simulink model "MC_R2_SFC_RELOJ_sin_antisway"  (R2025b)
settings: Solver=ode23t  StartTime=0.0  StopTime=600  MaxStep=T_s  RelTol=1e-4
InitFcn:
  | addpath(fileparts(get_param(bdroot,'FileName')),'-begin');
  | run(fullfile(fileparts(get_param(bdroot,'FileName')),'definir_buses_variadores.m'));
  | run(fullfile(fileparts(get_param(bdroot,'FileName')),'parametros_ganancias_cascada_29072026.m'));
  | run(fullfile(fileparts(get_param(bdroot,'FileName')),'configurar_modelo_final_hmi.m'));
  | run(fullfile(fileparts(get_param(bdroot,'FileName')),'configurar_parametros_variadores.m'));
  | Pvis.Ts_viz=0.04;Pvis.hmi.testDriver=@operador_medio_ciclo;
StopFcn:
  | cerrar_video_ensayo;
values from neighbouring files (symbols this model uses):
  MC_FF = struct('Ts',T_s,'gravity',g,'r_td',r_td,'i_t',i_t,'M_EQt',M_EQt,   'b_EQt',b_EQt,'Kx',K_x_cas,'Kp',K_pv_cas,'Ki',K_iv_cas,   'vmax',v_tmax,'amax',dv_tmax,'Imax',dv_tmax/K_iv_cas,   'r_hd',r_hd,'i_h',i_h,'M_EQh',M_EQh,'b_EQh',b_EQh,   'Khp',K_hp,'Khi',K_hi,'Khd',K_hd,'length0',l_hi,'swayOnTime',T_SW_on,   'swayFFRate',0.25,'observerWn',40.0,'observerZeta',1.0)    [configurar_parametros_variadores.m]
undefined symbols (not defined in the file or in its folder): b_cx, b_cy, b_hb, b_hEb, b_heq, b_t, b_tb, b_teq, b_tw, b_wu, g, H_c, HMI, i_h, i_t, J_heq, J_teq, K_cy, K_tw, k_wu, L_h0, l_hi, M_c_profile, M_s, M_t, nLevels0, omega_hmRATED, r_hd, r_td, slotBlock, T_hbMax, T_hEbMax, T_hmMax, T_s, T_s1, T_tbMax, T_tmMax, tau_hm, tau_tm, traj_duration, traj_x_start, traj_x_target, v_hmaxLoaded, v_hmaxUnloaded, x_tmax, x_tmin, Y_c0, Y_t0, Zbase
libraries: simulink x1, aerolibanimutils x1
(part 3 of 3)

== system MC_R2_SFC_RELOJ_sin_antisway/Planta/Subsistema carro/Modelo Freno Operacion Carro ==
  BRK_t : Inport
  omega_tm : Inport  Port=2
  Constant : Constant  Value=0
  Gain : Gain  Gain=-b_tb
  Saturation : Saturate  UpperLimit=T_tbMax  LowerLimit=-T_tbMax
  Switch : Switch  Criteria=u2 > Threshold  SaturateOnIntegerOverflow=off  InputSameDT=off
  T_tb : Outport
  wires:
  Saturation/1 -> Switch/3
  omega_tm/1 -> Gain/1
  Switch/1 -> T_tb/1
  Gain/1 -> Saturation/1
  Constant/1 -> Switch/1
  BRK_t/1 -> Switch/2

== system MC_R2_SFC_RELOJ_sin_antisway/Planta/Subsistema carro/Modulador de Torque Motor Drive Carro ==
  T_tm* : Inport
  Diferencia torque saturacion : Sum  Inputs=+-
  Gain : Gain  Gain=1/tau_tm
  Integrator : Integrator
  Saturation : Saturate  UpperLimit=T_tmMax  LowerLimit=-T_tmMax
  Sum : Sum  Inputs=|+-
  T_tm : Outport
  Delta torque limite : Outport  Port=2
  wires:
  Integrator/1 -> Sum/2, T_tm/1
  Gain/1 -> Integrator/1
  Sum/1 -> Gain/1
  Saturation/1 -> Sum/1, Diferencia torque saturacion/1  "T_tmlim*"
  T_tm*/1 -> Saturation/1, Diferencia torque saturacion/2
  Diferencia torque saturacion/1 -> Delta torque limite/1

== system MC_R2_SFC_RELOJ_sin_antisway/Planta/Subsistema izaje/Calculo longitud l_h ==
  note: $\dot{l}_h(t)=-\frac{r_{hd}}{2}\omega_{hd}(t)$
  omega_hd : Inport
  Gain : Gain  Gain=-r_hd/2
  Integrator : Integrator  InitialCondition=l_hi
  l_h : Outport
  dl_h : Outport  Port=2
  wires:
  Integrator/1 -> l_h/1  "l_h"
  omega_hd/1 -> Gain/1
  Gain/1 -> dl_h/1, Integrator/1  "dl_h"

== system MC_R2_SFC_RELOJ_sin_antisway/Planta/Subsistema izaje/Dinamica Tambor Izaje ==
  T_hEb : Inport
  T_hm : Inport  Port=2
  F_hw : Inport  Port=3
  T_hb : Inport  Port=4
  Gain1 : Gain  Gain=r_hd
  Gain2 : Gain  Gain=1/i_h
  Gain3 : Gain  Gain=1/J_heq
  Gain4 : Gain  Gain=b_heq
  Gain5 : Gain  Gain=1/i_h
  Integrator2 : Integrator
  Integrator3 : Integrator
  Sum1 : Sum  Inputs=+++--
  theta_hd : Outport
  omega_hd : Outport  Port=2
  wires:
  Gain3/1 -> Integrator2/1  "ddtheta_hd"
  Integrator2/1 -> omega_hd/1, Gain4/1, Integrator3/1  "omega_hd"
  Sum1/1 -> Gain3/1
  T_hb/1 -> Sum1/2
  T_hEb/1 -> Gain5/1  "T_hEb"
  Gain4/1 -> Sum1/5
  Gain5/1 -> Sum1/3
  T_hm/1 -> Sum1/1
  F_hw/1 -> Gain1/1
  Gain1/1 -> Gain2/1  "T_hdl"
  Gain2/1 -> Sum1/4
  Integrator3/1 -> theta_hd/1  "theta_hd"

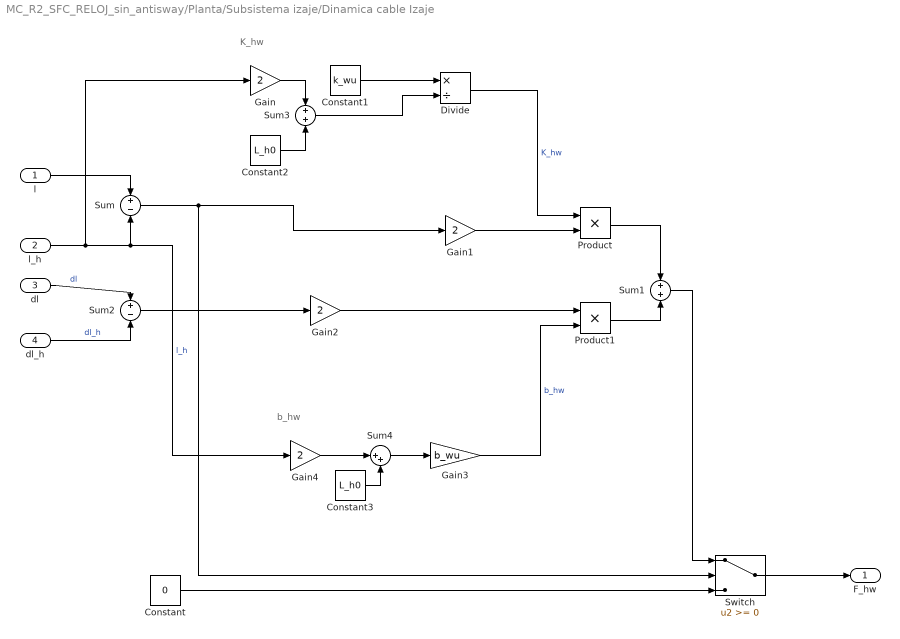
== system MC_R2_SFC_RELOJ_sin_antisway/Planta/Subsistema izaje/Dinamica cable Izaje ==
  note: b_hw
  note: K_hw
  l : Inport
  l_h : Inport  Port=2
  dl : Inport  Port=3
  dl_h : Inport  Port=4
  Constant : Constant  Value=0
  Constant1 : Constant  Value=k_wu
  Constant2 : Constant  Value=L_h0
  Constant3 : Constant  Value=L_h0
  Divide : Product  Inputs=*/
  Gain{,1..2,4} (4 alike) : Gain  Gain=2
  Gain3 : Gain  Gain=b_wu
  Product : Product
  Product1 : Product
  Sum : Sum  Inputs=+-
  Sum1 : Sum
  Sum2 : Sum  Inputs=+-
  Sum3 : Sum
  Sum4 : Sum  Inputs=|++
  Switch : Switch  SaturateOnIntegerOverflow=off  InputSameDT=off
  F_hw : Outport
  wires:
  Constant/1 -> Switch/3
  l/1 -> Sum/1
  l_h/1 -> Gain4/1, Sum/2, Gain/1  "l_h"
  Sum/1 -> Switch/2, Gain1/1
  Switch/1 -> F_hw/1
  Sum1/1 -> Switch/1
  Gain1/1 -> Product/2
  Product/1 -> Sum1/1
  Divide/1 -> Product/1  "K_hw"
  Gain3/1 -> Product1/2  "b_hw"
  dl/1 -> Sum2/1  "dl"
  dl_h/1 -> Sum2/2  "dl_h"
  Sum2/1 -> Gain2/1
  Gain2/1 -> Product1/1
  Product1/1 -> Sum1/2
  Sum3/1 -> Divide/2
  Constant1/1 -> Divide/1
  Constant2/1 -> Sum3/2
  Gain/1 -> Sum3/1
  Gain4/1 -> Sum4/1
  Sum4/1 -> Gain3/1
  Constant3/1 -> Sum4/2

== system MC_R2_SFC_RELOJ_sin_antisway/Planta/Subsistema izaje/Modelo Freno Emergencia de Izaje(Eje lento) ==
  omega_hd : Inport
  BRK_hE : Inport  Port=2
  Constant : Constant  Value=0
  Gain : Gain  Gain=-b_hEb
  Saturation : Saturate  UpperLimit=T_hEbMax  LowerLimit=-T_hEbMax
  Switch : Switch  Criteria=u2 > Threshold  SaturateOnIntegerOverflow=off  InputSameDT=off
  T_hEb : Outport
  wires:
  Saturation/1 -> Switch/3
  omega_hd/1 -> Gain/1
  Switch/1 -> T_hEb/1
  Gain/1 -> Saturation/1
  Constant/1 -> Switch/1
  BRK_hE/1 -> Switch/2

== system MC_R2_SFC_RELOJ_sin_antisway/Planta/Subsistema izaje/Modelo Freno Operacion de Izaje(Eje Rapido) ==
  BRK_h : Inport
  omega_hm : Inport  Port=2
  Constant : Constant  Value=0
  Gain : Gain  Gain=-b_hb
  Saturation : Saturate  UpperLimit=T_hbMax  LowerLimit=-T_hbMax
  Switch : Switch  Criteria=u2 > Threshold  SaturateOnIntegerOverflow=off  InputSameDT=off
  T_hb : Outport
  wires:
  Saturation/1 -> Switch/3
  omega_hm/1 -> Gain/1
  Switch/1 -> T_hb/1
  Gain/1 -> Saturation/1
  Constant/1 -> Switch/1
  BRK_h/1 -> Switch/2

== system MC_R2_SFC_RELOJ_sin_antisway/Planta/Subsistema izaje/Modulador de Torque Motor Drive Izaje ==
  T_hm* : Inport
  omega_hm : Inport  Port=2
  Calculo Torque Limite : Subsystem
  Gain : Gain  Gain=1/tau_hm
  Gain1 : Gain  Gain=-1
  Integrator : Integrator
  Saturation Dynamic : simulink/Discontinuities/Saturation Dynamic  OutMin=[]  OutMax=[]  OutDataTypeStr=Inherit: Same as second input  OutDataType=fixdt(1, 16)  OutScaling=2^-10  DoSatur=off
  Sum : Sum  Inputs=|+-
  T_hm : Outport
  wires:
  Gain/1 -> Integrator/1
  Sum/1 -> Gain/1
  Integrator/1 -> T_hm/1, Sum/2
  Saturation Dynamic/1 -> Sum/1  "Thm_sat"
  T_hm*/1 -> Saturation Dynamic/2
  omega_hm/1 -> Calculo Torque Limite/1(omega_hm)
  Calculo Torque Limite/1(T_hmMax) -> Gain1/1, Saturation Dynamic/1
  Gain1/1 -> Saturation Dynamic/3

== system MC_R2_SFC_RELOJ_sin_antisway/Planta/Subsistema izaje/Modulador de Torque Motor Drive Izaje/Calculo Torque Limite ==
  omega_hm : Inport
  Abs omega : Abs  SaturateOnIntegerOverflow=off
  Constant2 : Constant
  Divide : Product  Inputs=*/
  Gain1 : Gain  Gain=T_hmMax
  Min : MinMax  Inputs=2
  Proteccion omega cero : Saturate  UpperLimit=inf  LowerLimit=1e-6
  Square : Math  Operator=square
  omega_hmRATED : Constant  Value=omega_hmRATED
  T_hmMax : Outport
  wires:
  omega_hmRATED/1 -> Divide/1
  Gain1/1 -> T_hmMax/1  "T_hmMax"
  Min/1 -> Gain1/1
  Constant2/1 -> Min/2
  Square/1 -> Min/1
  Divide/1 -> Square/1
  omega_hm/1 -> Abs omega/1
  Abs omega/1 -> Proteccion omega cero/1
  Proteccion omega cero/1 -> Divide/2

== stateflow chart MC_R2_SFC_RELOJ_sin_antisway/PICK // PLACE ==
  state INICIO
    entry:
    evento_cambio = false;
    tipo_evento = 0;
    slot_evento = -1;
    slot_mem = -1;
    carga_tomada = TLK;
  state VACIO1
    during:
    evento_cambio = false;
    tipo_evento = 0;
    slot_evento = -1;
    carga_tomada = 0;
  state PRE_PLACE
    during:
    evento_cambio = false;
    tipo_evento = 0;
    slot_evento = -1;
    carga_tomada = 1;
  state CARGADO1
    during:
    evento_cambio = false;
    tipo_evento = 0;
    slot_evento = -1;
    carga_tomada = 1;
  state PRE_PICK
    during:
    evento_cambio = false;
    tipo_evento = 0;
    slot_evento = -1;
    carga_tomada = 0;
  (default) -> ? [commented out]
  (default) -> ? [commented out] : [slot_ok && TLK == 1 && tension && ~contacto && v_yl > -0.05]{slot_evento = k_slot;}
  (default) -> ? [commented out] : [slot_ok && TLK == 0 && ~tension && contacto && abs(v_yl) < 0.05]{slot_evento = k_slot;}
  (default) -> ? [commented out] : [true]
  (default) -> INICIO
  INICIO -> VACIO1 [order 1] : [TLK==0]
  INICIO -> CARGADO1 [order 2] : [TLK ==1]
  PRE_PLACE -> VACIO1 [order 2] : [slot_ok && TLK == 0 && contacto]{evento_cambio = true; tipo_evento = 2; slot_evento = slot_mem;}
  CARGADO1 -> PRE_PLACE : [slot_ok && TLK == 1 && contacto && abs(v_yl) < 0.05]{slot_mem = k_slot;}
  PRE_PICK -> VACIO1 [order 1] : [~slot_ok || (~contacto && TLK == 0)]{slot_mem = -1;}
  PRE_PLACE -> CARGADO1 [order 1] : [TLK == 1 && tension && ~contacto && v_yl > 0.05]{slot_mem = -1;}
  VACIO1 -> PRE_PICK : [slot_ok && contacto && TLK == 0]{slot_mem = k_slot;}
  PRE_PICK -> CARGADO1 [order 2] : [slot_ok && TLK == 1 && tension && ~contacto && v_yl > 0.05]{evento_cambio = true; tipo_evento = 1; slot_evento = slot_mem;}
  data: TLK input; k_slot input; slot_ok input; v_yl input; evento_cambio output; tipo_evento output; slot_evento output int32; contacto input; tension input; slot_mem local int32; carga_tomada output

== matlab function MC_R2_SFC_RELOJ_sin_antisway/Histeresis_F_hw ==
  data: F_hw input; tension output
function tension = tension_hist_Fhw(F_hw)
% Histeresis física para detectar "cable cargado" a partir de F_hw [N].
% Basada en fracciones del peso mínimo (spreader + contenedor vacío).

% --- Parámetros físicos ---
g = 9.81;
M_s    = 15000;   % kg
M_cmin = 2000;    % kg

Wmin = (M_s + M_cmin) * g;     % N  ~ 167 kN

% --- Umbrales con histéresis ---
Fhw_on  = 0.21 * Wmin;         % ~ 35 kN (cable claramente cargado)
Fhw_off = 0.09 * Wmin;         % ~ 15 kN (cable claramente descargado)

% --- Estado persistente ---
persistent t
if isempty(t)
    t = false;
end

% --- Lógica de histéresis ---
if ~t
    if F_hw > Fhw_on
        t = true;
    end
else
    if F_hw < Fhw_off
        t = false;
    end
end

tension = t;
end

== matlab function MC_R2_SFC_RELOJ_sin_antisway/Histeresis_contacto ==
  data: F_cy input; contacto output
function contacto = contacto_hist_Fcy(F_cy)
% Histeresis física para detectar contacto a partir de F_cy [N].
% Basada en fracciones del peso mínimo (spreader + contenedor vacío).

% --- Parámetros físicos ---
g = 9.81;
M_s    = 15000;   % kg
M_cmin = 2000;    % kg

Wmin = (M_s + M_cmin) * g;     % N  ~ 167 kN

% --- Umbrales con histéresis ---
Fcy_on  = 0.03  * Wmin;        % ~ 5 kN (entra a contacto)
Fcy_off = 0.012 * Wmin;        % ~ 2 kN (sale de contacto)

% --- Estado persistente ---
persistent c
if isempty(c)
    c = false;
end

% --- Lógica de histéresis ---
if ~c
    if F_cy > Fcy_on
        c = true;
    end
else
    if F_cy < Fcy_off
        c = false;
    end
end

contacto = c;
end

== matlab function MC_R2_SFC_RELOJ_sin_antisway/slot_x_l ==
  data: x_l input; k_slot output; slot_ok output; slotBlock input
function [k_slot, slot_ok] = xl_a_slot(x_l, slotBlock)
%#codegen

x0 = -30.0;
slotWidth = 2.44;
Nslots = int32(length(slotBlock));

k = int32(1) + int32(floor((x_l - x0) / slotWidth));

if (k < 1) || (k > Nslots)
    k_slot = int32(-1);
    slot_ok = false;
else
    k_slot = k;
    slot_ok = ~slotBlock(k_slot);
end

end

== matlab function MC_R2_SFC_RELOJ_sin_antisway/Actualizar_Yc/update_perfil_std ==
  data: nLevels input; nLevels_new output; tipo_evento input; slot_evento input; Y_c output; Zbase input; slotBlock input; h_std input
function [nLevels_new, Y_c] = update_profile_std(nLevels, tipo_evento, slot_evento, Zbase, slotBlock, h_std)
% UPDATE_PROFILE_STD
% Actualiza el perfil discreto de obstáculos.
% Convención:
%   Y_c(k)       = altura absoluta física del tope del obstáculo.
%   nLevels(k)  = cantidad de containers en el slot k.
%   Zbase(k)    = base física absoluta del slot k.
%   slotBlock(k)= true si el slot no es operable.
%
% tipo_evento:
%   0 = NONE
%   1 = PICK
%   2 = PLACE

Nslots = int32(length(nLevels));

nLevels_new = nLevels;

slot = int32(slot_evento);

slot_ok = (slot >= 1) && (slot <= Nslots) && (~slotBlock(slot));

if slot_ok
    if tipo_evento == 1
        nLevels_new(slot) = max(nLevels_new(slot) - 1, 0);

    elseif tipo_evento == 2
        nLevels_new(slot) = nLevels_new(slot) + 1;
    end

end

Y_c = Zbase + double(nLevels_new) * h_std;

% En slots bloqueados no se codifica bloqueo dentro de Y_c.
% Se deja una altura neutral coherente con Zbase.
Y_c(slotBlock) = Zbase(slotBlock);

end

== stateflow chart MC_R2_SFC_RELOJ_sin_antisway/Trayectoria ==
  settings: updateMethod=DISCRETE  sampleTime=T_s  description=Generador parametrico de septimo orden. Mantiene continuas x, v, a y jerk y conserva la interfaz original.
  state Perfil_suave
    during:
    tau = elapsed/traj_duration;
    if tau > 1
    tau = 1;
    end
    delta_x = traj_x_target-traj_x_start;
    sigma = 35*tau^4-84*tau^5+70*tau^6-20*tau^7;
    dsigma = 140*tau^3-420*tau^4+420*tau^5-140*tau^6;
    d2sigma = 420*tau^2-1680*tau^3+2100*tau^4-840*tau^5;
    d3sigma = 840*tau-5040*tau^2+8400*tau^3-4200*tau^4;
    x_act = traj_x_start+delta_x*sigma;
    v_act = delta_x*dsigma/traj_duration;
    a_act = delta_x*d2sigma/(traj_duration^2);
    j_act = delta_x*d3sigma/(traj_duration^3);
    elapsed = elapsed+T_s;
  state Objetivo
    entry:
    x_act = traj_x_target;
    v_act = 0;
    a_act = 0;
    j_act = 0;
  state Esperando
    entry:
    elapsed = 0;
    x_act = traj_x_start;
    v_act = 0;
    a_act = 0;
    j_act = 0;
  (default) -> Esperando
  Perfil_suave -> Objetivo : [elapsed >= traj_duration]
  Esperando -> Perfil_suave : [iniciar == 1]
  data: j_k function_output; v_max function_input; a_max function_input; j_max function_input; j_min function_input; v_k function_input; a_k function_input; d_k function_output; fa_min function_input; a_min function_input; j_max function_input; j_min function_input; a_k function_input; a_1 function_input; v_k function_input; v_1 function_input; T_j2a function_output; T_j2b function_output; T_d function_output; j_k function_output; j_min function_input; j_max function_input; k function_input; k_d function_input; T_s function_input; T_d function_input; T_j2a function_input; T_j2b function_input; iniciar input double =0; v_act output double =0; x_act output double =0; a_act output double =0; j_act output double =0; traj_x_start parameter double; traj_x_target parameter double; traj_duration parameter double; T_s parameter double; elapsed local double =0; tau local double =0; delta_x local double =0; sigma local double =0; dsigma local double =0; d2sigma local double =0; d3sigma local double =0
  function j_k=calculo_jerk(v_max, a_max, j_max, j_min, v_k, a_k):
    | function j_k=calculo_jerk(v_max, a_max, j_max, j_min, v_k, a_k)
    | 
    | if ((v_k-(a_k^2)/(2*j_min))<v_max)&&(a_k<a_max)
    |     j_k = j_max;
    | elseif ((v_k-(a_k^2)/(2*j_min))<v_max)&&(a_k>=a_max)
    |     j_k = 0;
    | elseif ((v_k-(a_k^2)/(2*j_min))>=v_max)&&(a_k>0)
    |     j_k = j_min;
    | elseif ((v_k-(a_k^2)/(2*j_min))>=v_max)&&(a_k<=0)
    |     j_k = 0;
    | else
    |     j_k = 0;
    | end
  function [d_k, T_j2a, T_j2b, T_d]=calculo_dist_frenado(fa_min, a_min, j_max, j_min, a_k, a_1, v_k, v_1):
    | function [d_k, T_j2a, T_j2b, T_d]=calculo_dist_frenado(fa_min, a_min, j_max, j_min, a_k, a_1, v_k, v_1)
    | 
    | if fa_min==1
    |     T_j2a = (a_min-a_k)/j_min;
    |     T_j2b = (a_1-a_min)/j_max;
    |     T_d = (v_1-v_k)/a_min + T_j2a*(a_min-a_k)/(2*a_min) + T_j2b*(a_min-a_1)/(2*a_min);
    | else
    |     T_j2a = -a_k/j_min + sqrt((j_max-j_min)*(a_k^2*j_max-j_min*(a_1^2+2*j_max*(v_k-v_1))))/(j_min*(j_min-j_max));
    |     T_j2b = a_1/j_max + sqrt((j_max-j_min)*(a_k^2*j_max-j_min*(a_1^2+2*j_max*(v_k-v_1))))/(j_max*(j_max-j_min));
    |     T_d = T_j2a + T_j2b;
    | end
    | 
    | d_k = (a_k*T_d^2)/2 + (j_min*T_j2a*((3*T_d^2)-(3*T_d*T_j2a)+(T_j2a^2))+j_max*T_j2b^3)/6 + T_d*v_k;
  function j_k=calculo_jerk_des(j_min, j_max, k, k_d, T_s, T_d, T_j2a, T_j2b):
    | function j_k=calculo_jerk_des(j_min, j_max, k, k_d, T_s, T_d, T_j2a, T_j2b)
    | if ((k-k_d)>=0)&&((k-k_d)<(T_j2a/T_s))
    |     j_k = j_min;
    | elseif ((k-k_d)>=(T_j2a/T_s))&&((k-k_d)<((T_d-T_j2b)/T_s))
    |     j_k = 0;
    | elseif ((k-k_d)>=((T_d-T_j2b)/T_s))&&((k-k_d)<=(T_d/T_s))
    |     j_k = j_max;
    | else
    |     j_k = 0;
    | end

== matlab function MC_R2_SFC_RELOJ_sin_antisway/Nivel 0 - Seguridad/Sensores de seguridad ==
  data: xT input; LST_MINU output; vT input; yH input; vH input; LST_MAXU output; LSH_MINU output; LSH_MAXU output; VH_MAX output
function [LST_MINU,LST_MAXU,LSH_MINU,LSH_MAXU,VH_MAX] = detectar(xT,vT,yH,vH)
%#codegen
LST_MINU = (xT <= -30.5) || (vT <= -4.6);
LST_MAXU = (xT >=  50.5) || (vT >=  4.6);
LSH_MINU = yH <= -20.5;
LSH_MAXU = yH >=  40.5;
VH_MAX = abs(vH) >= 3.45;
end

== matlab function MC_R2_SFC_RELOJ_sin_antisway/MASS_latch_pick ==
  settings: updateMethod=DISCRETE  sampleTime=0.001
  data: profileMass input; mass output; loaded input
function mass = latchPickedMass(profileMass,loaded)
%#codegen
persistent heldMass previousLoaded
if isempty(heldMass)
    heldMass=0.0; previousLoaded=false;
end
isLoaded=loaded>=0.5;
if isLoaded && ~previousLoaded
    heldMass=max(0.0,profileMass);
elseif ~isLoaded
    heldMass=0.0;
end
mass=heldMass; previousLoaded=isLoaded;
end

== matlab function MC_R2_SFC_RELOJ_sin_antisway/Motion Controller/MC Izaje ==
  settings: updateMethod=DISCRETE  sampleTime=T_s
  data: s input Bus: MCFF_Sensors; torque output; r input Bus: MCFF_References; est input Bus: MCFF_HoistState; p input Bus: MCFF_Parameters; d output Bus: MCFF_HoistDiagnostics
function [torque,d]=fcn(s,r,est,p)
%#codegen
% Variador de izaje. No implementa ninguna funcion del automata.
[torque,ev,z1,z2,P,D,I,ff]=controlador_izaje_mc_r2( ...
 s.force,-r.hoistVelocityRef,est.lengthRate,-r.hoistAccelerationRef,p);
d=struct('torque_izaje_consigna_controlador',torque,'mc_hoist_velocity_error',ev, ...
 'mc_hoist_integral1',z1,'mc_hoist_integral2',z2,'mc_hoist_P',P, ...
 'mc_hoist_D',D,'mc_hoist_I',I,'mc_hoist_FF',ff);
end
function [torque,errorVelocity,z1,z2,pTerm,dTerm,iTerm,ff]= ...
 controlador_izaje_mc_r2(force,vRef,vMeasured,aRef,p)
%#codegen
% Doble integracion Tustin de R2, sin seleccion por modo ni AW adicional.
persistent firstIntegral secondIntegral previousError previousFirst
if isempty(firstIntegral)
 firstIntegral=0.0;secondIntegral=0.0;previousError=0.0;previousFirst=0.0;
end
errorVelocity=vRef-vMeasured;
firstIntegral=(p.Ts/2)*(previousError+errorVelocity)+firstIntegral;
secondIntegral=(p.Ts/2)*(previousFirst+firstIntegral)+secondIntegral;
z1=firstIntegral;z2=secondIntegral;
pTerm=p.Khp*z1;dTerm=p.Khd*errorVelocity;iTerm=p.Khi*z2;
feedback=(iTerm+pTerm)+dTerm;
forceTerm=(-p.r_hd/p.i_h)*force;
ff=(-p.r_hd/p.i_h)*(p.M_EQh*aRef+p.b_EQh*vRef);
torque=ff+(feedback-forceTerm);
previousError=errorVelocity;previousFirst=firstIntegral;
end

== matlab function MC_R2_SFC_RELOJ_sin_antisway/Motion Controller/MC Carro ==
  settings: updateMethod=DISCRETE  sampleTime=T_s
  data: s input Bus: MCFF_Sensors; torque output; r input Bus: MCFF_References; c input Bus: MCFF_Commands; drive input Bus: MCFF_DriveFeedback; est input Bus: MCFF_TrolleyState; hoist input Bus: MCFF_HoistState; p input Bus: MCFF_Parameters; sw output; d output Bus: MCFF_TrolleyDiagnostics
function [torque,sw,d]=fcn(s,r,c,drive,est,hoist,p)
%#codegen
% Variador de carro. Estimaciones recibidas del estimador interno del MC.
persistent ff gain
if isempty(gain),ff=0.0;gain=0.0;end
omega=est.omegaDrum;
k=2.0*sqrt(p.gravity*hoist.length); anticipationGain=2.0*sqrt(9.80665*max(1.0,hoist.length));
thetaEff=double(c.E)*s.theta;
feedback=k*(thetaEff-0.0);
thetaRef=atan2(-r.aRef,p.gravity);
if ~c.E || ~c.brakeOpen
 ff=0.0;gain=0.0;sw=0.0;feedbackUsed=0.0;anticipationUsed=0.0;
else
 gain=min(1.0,gain+max(1e-6,p.Ts)/p.swayOnTime);
 target=-anticipationGain*thetaRef;
 h=max(1e-6,p.Ts);
 ff=ff+min(p.swayFFRate*h,max(-p.swayFFRate*h,target-ff));
 anticipation=ff;
 feedbackUsed=gain*feedback;anticipationUsed=gain*anticipation;
 sw=min(3.2,max(-3.2,feedbackUsed+anticipationUsed));
end
swCalculated=sw;
sw=0*swCalculated;
vBase=(r.vRef+sw)+r.swTransfer;
[torque,vRaw,vCmd,vObs,I,pTerm,iTerm,aRaw,aCmd,ev,deltaA,deltaAPrevious, ...
 deltaATorque,deltaATotal,awCorrection,uI]=controlador_carro_mc_r2( ...
 s.force,omega,vBase,r.xRef,r.aRef,est.x,s.theta,drive.deltaTorqueDelayed,p);
d=struct('diag_torque_unsat',torque,'diag_vcmd',vRaw,'diag_vcmd_applied',vCmd, ...
 'diag_vobs',vObs,'diag_integral',I,'diag_p',pTerm,'diag_i',iTerm,'diag_acmd',aRaw, ...
 'diag_acmd_applied',aCmd,'diag_ev',ev,'aw_delta_a_limite',deltaA, ...
 'aw_delta_a_limite_memoria',deltaAPrevious,'aw_delta_a_torque',deltaATorque, ...
 'aw_delta_a_total',deltaATotal,'aw_correccion_integrador',awCorrection, ...
 'mc_integrator_input',uI,'antisway_correccion_aplicada',sw, ...
 'sw_feedback_comun',feedbackUsed,'sw_anticipacion_comun',anticipationUsed, ...
 'sw_habilitacion_comun',gain,'diag_sw_unsat',feedbackUsed+anticipationUsed,'diag_sw_gain',k, ...
 'angulo_referencia',thetaRef,'diag_aff',r.aRef,'diag_xref_input',r.xRef, ...
 'diag_vref_input',r.vRef,'diag_aref_input',r.aRef,'diag_xencoder',est.x, ...
 'diag_omega_observer',omega,'diag_theta_medida',s.theta,'diag_theta_eff',thetaEff, ...
 'diag_brake_supervisor',double(c.brakeOpen),'ensayo_vcmd_sum',vBase,'ensayo_sw_limitada',swCalculated);
end
function [torque,vRaw,vCmd,vObs,I,pTerm,iTerm,aRaw,aCmd,ev, ...
 deltaA,deltaAPrevious,deltaATorque,deltaATotal,awCorrection,uI]= ...
 controlador_carro_mc_r2(force,omega,vBase,xRef,aRef,x,theta,deltaTorque,p)
%#codegen
% N2 de R2: PI Tustin limitado, AW de aceleracion y torque con demora 1 ms.
% El regulador no recibe modo, enable de eje ni reset; N0 autoriza el par.
persistent integralState previousDeltaA
if isempty(integralState)
 integralState=0.0;previousDeltaA=0.0;
end
vObs=p.r_td*omega;
vRaw=vBase+p.Kx*(xRef-x);
vCmd=min(p.vmax,max(-p.vmax,vRaw));
ev=vCmd-vObs;
deltaAPrevious=previousDeltaA;
deltaATorque=(p.i_t/(p.r_td*p.M_EQt))*deltaTorque;
deltaATotal=deltaAPrevious+deltaATorque;
awCorrection=(1/p.Ki)*deltaATotal;
uI=ev+awCorrection;
% IC=0 es el estado X; la salida incluye el medio paso de entrada actual.
I=min(p.Imax,max(-p.Imax,integralState+p.Ts/2*uI));
% El bloque original limita salida Y y estado X por separado en Tustin.
% Esto permite salir del limite en el primer medio paso de signo contrario.
integralState=min(p.Imax,max(-p.Imax,I+p.Ts/2*uI));
pTerm=p.Kp*ev;iTerm=p.Ki*I;
aRaw=aRef+(pTerm+iTerm);
aCmd=min(p.amax,max(-p.amax,aRaw));
deltaA=aCmd-aRaw;
% Conservar la estructura de operaciones del Computed Torque de R2.
friction=(p.b_EQt/p.M_EQt)*vObs;
horizontal=(2/p.M_EQt)*(force*sin(theta));
torque=((p.r_td*p.M_EQt)/p.i_t)*((friction+aCmd)-horizontal);
previousDeltaA=deltaA;
end

== matlab function MC_R2_SFC_RELOJ_sin_antisway/Motion Controller/Estimadores ==
  settings: updateMethod=DISCRETE  sampleTime=T_s
  data: s input Bus: MCFF_Sensors; cart output Bus: MCFF_TrolleyState; p input Bus: MCFF_Parameters; hoist output Bus: MCFF_HoistState
function [cart,hoist]=fcn(s,p)
%#codegen
% Dos observadores Tustin de encoders, independientes de referencias y modos.
persistent qt wt qh wh previousT previousH started
if isempty(qt)
 qt=0.0;wt=0.0;qh=0.0;wh=0.0;previousT=0.0;previousH=0.0;started=false;
end
ut=s.motorAngleT/p.i_t;uh=s.motorAngleH/p.i_h;
if started
 [qt,wt]=actualizar_observador_encoder(qt,wt,previousT,ut,p);
 [qh,wh]=actualizar_observador_encoder(qh,wh,previousH,uh,p);
else
 started=true;
end
previousT=ut;previousH=uh;
cart=struct('x',p.r_td*ut,'omegaDrum',wt,'velocity',p.r_td*wt,'observerAngle',qt);
hoist=struct('length',p.length0-(p.r_hd/2)*uh,'lengthRate',(p.r_hd/(-2))*wh, ...
 'omegaDrum',wh,'observerAngle',qh);
end
function [qNext,wNext]=actualizar_observador_encoder(q,w,uPrevious,u,p)
%#codegen
% Trapezoidal: x[n]=Ad*x[n-1]+Bd*(u[n-1]+u[n]).
% La primera muestra y la IC=0 se manejan en el propietario del estado.
qNext=(p.obsA11*q+p.obsA12*w)+p.obsB1*(uPrevious+u);
wNext=(p.obsA21*q+p.obsA22*w)+p.obsB2*(uPrevious+u);
end

== matlab function MC_R2_SFC_RELOJ_sin_antisway/Consigna Izaje ==
  data: lh_ref output; dlh_ref output; t input; ddlh_ref output; done output
function [lh_ref, dlh_ref, ddlh_ref, done] = trayectoria_lh_quintica(t)
%#codegen
% Trayectoria suave para longitud de cable l_h.
%
% Tramo 1:
%   l_h: 20 m -> 34 m
%   inicia en t = 15 s
%
% Tramo 2:
%   l_h: 34 m -> 29 m
%   inicia en t = 45 s
%
% Salidas:
%   lh_ref   : referencia de longitud [m]
%   dlh_ref  : velocidad de longitud [m/s]
%   ddlh_ref : aceleración de longitud [m/s^2]
%   done     : true cuando terminó toda la secuencia

% Parámetros tramo 1: bajar / desenrollar
lh0_1   = 20.0;     % [m]
lhf_1   = 26.5;     % [m]
t_ini_1 = 15.0;     % [s]
Tmov_1  = 12.0;     % [s]

% Parámetros tramo 2: subir / enrollar 5 m
lh0_2   = lhf_1;    % [m]
lhf_2   = lhf_1 - 5.0;  % [m]
t_ini_2 = 28.0;     % [s]
Tmov_2  = 8.0;      % [s]

% Antes del primer movimiento
if t < t_ini_1
    lh_ref   = lh0_1;
    dlh_ref  = 0.0;
    ddlh_ref = 0.0;
    done     = false;
    return;
end

% Tramo 1
if t < t_ini_1 + Tmov_1
    [lh_ref, dlh_ref, ddlh_ref] = tramo_quintico(t, t_ini_1, Tmov_1, lh0_1, lhf_1);
    done = false;
    return;
end

% Espera entre tramo 1 y tramo 2
if t < t_ini_2
    lh_ref   = lhf_1;
    dlh_ref  = 0.0;
    ddlh_ref = 0.0;
    done     = false;
    return;
end

% Tramo 2
if t < t_ini_2 + Tmov_2
    [lh_ref, dlh_ref, ddlh_ref] = tramo_quintico(t, t_ini_2, Tmov_2, lh0_2, lhf_2);
    done = false;
    return;
end

% Después de terminar todo
lh_ref   = lhf_2;
dlh_ref  = 0.0;
ddlh_ref = 0.0;
done     = true;

end

function [lh, dlh, ddlh] = tramo_quintico(t, t_ini, Tmov, lh0, lhf)
% Trayectoria quintica normalizada entre lh0 y lhf.

tau = (t - t_ini) / Tmov;

s   = 10*tau^3 - 15*tau^4 + 6*tau^5;
ds  = 30*tau^2 - 60*tau^3 + 30*tau^4;
dds = 60*tau - 180*tau^2 + 120*tau^3;

Dlh = lhf - lh0;

lh   = lh0 + Dlh * s;
dlh  = Dlh * ds / Tmov;
ddlh = Dlh * dds / (Tmov^2);

end
